simulink model "prueba"  (R2017b)
settings: Solver=VariableStepAuto  StartTime=0.0  StopTime=10.0  RelTol=1e-3
settings Model: Creator=jesusoroya  LastModifiedBy=jesusoroya

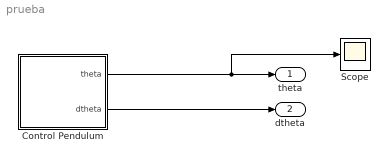
== system prueba ==
  Control Pendulum : Subsystem  mask{g=9.8, L=2, beta=1, theta0=2, dtheta0=0}
  Scope : Scope
  theta : Outport
  dtheta : Outport  Port=2
  wires:
  Control Pendulum/1(theta) -> Scope/1, theta/1
  Control Pendulum/2(dtheta) -> dtheta/1

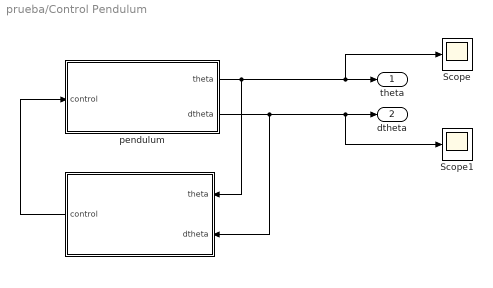
== system prueba/Control Pendulum ==
  " " : MATLAB Function  TreatAsAtomicUnit=on
  Scope : Scope
  Scope1 : Scope
  pendulum : Subsystem
  theta : Outport
  dtheta : Outport  Port=2
  wires:
  pendulum/1(theta) -> Scope/1, theta/1, " "/1(theta)
  " "/1(control) -> pendulum/1(control)
  pendulum/2(dtheta) -> Scope1/1, dtheta/1, " "/2(dtheta)

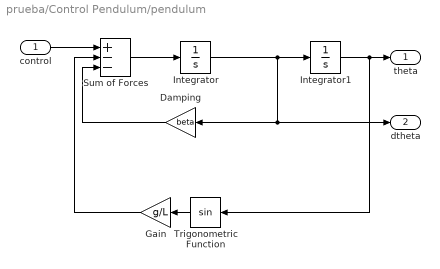
== system prueba/Control Pendulum/pendulum ==
  control : Inport
  Damping : Gain  Gain=beta
  Gain : Gain  Gain=g/L
  Integrator : Integrator  InitialCondition=theta0
  Integrator1 : Integrator  InitialCondition=dtheta0
  Sum of Forces : Sum  Inputs=+--
  Trigonometric Function : Trigonometry
  theta : Outport
  dtheta : Outport  Port=2
  wires:
  Integrator/1 -> dtheta/1, Damping/1, Integrator1/1
  Gain/1 -> Sum of Forces/2
  Integrator1/1 -> Trigonometric Function/1, theta/1
  Trigonometric Function/1 -> Gain/1
  control/1 -> Sum of Forces/1
  Sum of Forces/1 -> Integrator/1
  Damping/1 -> Sum of Forces/3

== matlab function prueba/Control Pendulum/  ==
  data: theta input; control output; dtheta input
function control = ControlMethod(theta,dtheta)

    
    control = 1;

    %%

end

function result = Jfunctional(theta,dtheta)
   E  = (1/2)*m*l^2*dtheta0^2 + m*g*l(1-cos(theta0));
   Et = (1/2)*m*l^2*dtheta^2 + m*g*l(1-cos(theta));
end
